simulink model "VTOLAutopilotController"  (R2025a)
settings: configuration reference "VTOLConfiguration" (kept outside this file)
undefined symbols (not defined in the file): Back_Transition_Rate, const, control, controlParams, ControlSampleTime, CriticalTiltAngle, DiscIntNeverNeededParam, dspblkCoreblockFVToolHelper, Fading_time, flightState, FSState, FWControlParams, FWTrimSpeed, gcbh, HoverMission, ReferenceFilterDen, ReferenceFilterNum, tilt_max, tiltIni, TransitioncontrolGains, uavParam, uavParams, VTOLcontrolGains, w_trim, WindDownRate
libraries: simulink x43, slpidlib x35, uavalgslib x7, simulink_extras x1
(part 1 of 8)
settings Model: DataDictionary=VTOLDynamicsData.sldd  PauseTimes=447  Creator=The MathWorks, Inc.  LastModifiedBy=mhcho
settings ConfigSetRef: SourceName=VTOLConfiguration

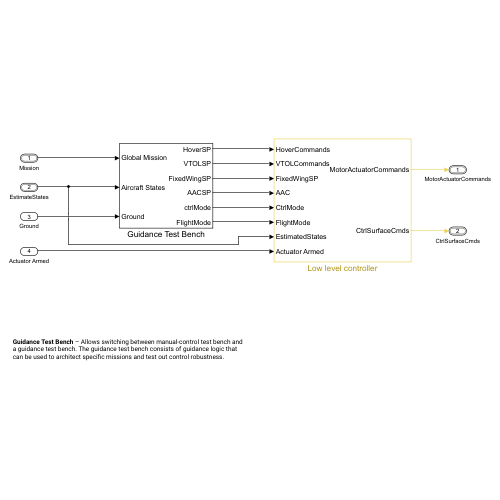
[thumbnail: Simulink's stored preview of the top-level diagram]
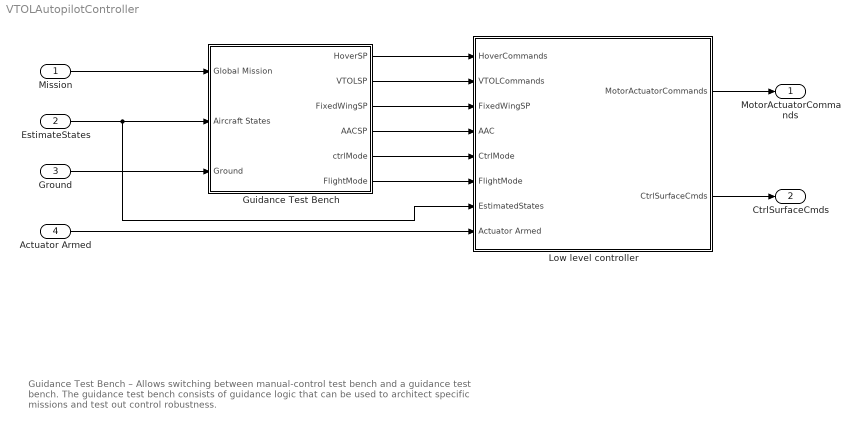
== system VTOLAutopilotController ==
  note: Guidance Test Bench – Allows switching between manual-control test bench and a guidance test bench. The guidance test bench consists of guidance logic that can be used to architect specific missions and test out control robustness.
  Mission : Inport  OutDataTypeStr=Bus: doubleUavPathManager  PortDimensions=length(HoverMission)  SampleTime=0.005  BusOutputAsStruct=on
  EstimateStates : Inport  Port=2  OutDataTypeStr=Bus: stateBus  BusOutputAsStruct=on
  Ground : Inport  Port=3  SampleTime=0.005
  Actuator Armed : Inport  Port=4
  Guidance Test Bench : Subsystem
  Low level controller : Subsystem
  MotorActuatorCommands : Outport  OutDataTypeStr=Bus: RotorCtrlBus  BusOutputAsStruct=on
  CtrlSurfaceCmds : Outport  Port=2  OutDataTypeStr=Bus: FixedWingCtrlBus  BusOutputAsStruct=on
  wires:
  Guidance Test Bench/1(HoverSP) -> Low level controller/1(HoverCommands)
  Guidance Test Bench/4(AACSP) -> Low level controller/4(AAC)
  Guidance Test Bench/6(FlightMode) -> Low level controller/6(FlightMode)
  Guidance Test Bench/5(ctrlMode) -> Low level controller/5(CtrlMode)
  EstimateStates/1 -> Low level controller/7(EstimatedStates), Guidance Test Bench/2(Aircraft States)
  Low level controller/1(MotorActuatorCommands) -> MotorActuatorCommands/1
  Mission/1 -> Guidance Test Bench/1(Global Mission)
  Guidance Test Bench/3(FixedWingSP) -> Low level controller/3(FixedWingSP)
  Low level controller/2(CtrlSurfaceCmds) -> CtrlSurfaceCmds/1
  Ground/1 -> Guidance Test Bench/3(Ground)
  Actuator Armed/1 -> Low level controller/8(Actuator Armed)
  Guidance Test Bench/2(VTOLSP) -> Low level controller/2(VTOLCommands)

== system VTOLAutopilotController/Guidance Test Bench ==
  note: Set control type. In the project shortcut, choose between:
      | 1. Manual control by selecting Manual Mode under Hover and open the subsystem to manually control the UAV in hover mode.
      | 2. Guidance testbench with prebuilt mission by selecting Guidance Mod e in the project shortcut.
  Global Mission : Inport
  Aircraft States : Inport  Port=2
  Ground : Inport  Port=3
  ControlType : Subsystem  Variant=on  VariantControl=Choice
  Variant Subsystem : Subsystem  Variant=on
      settings: PortSchema="{\"entries\":[{\"content\":{\"sides\":[{\"content\":{\"connectorIds\":[\"In1\"]},\"type\":\"ConnectorPlacement.EquallySpacedRectSide\",\"uuid\":\"9fdb7eb7-bc98-4ae8-8dfe-5c3a3cbe5bd4\"},{\"content\":{\"connectorIds\":[\"In2\",\"In3\",\"In4\",\"In5\"],\"side\":\"RIGHT\"},\"type\":\"ConnectorPlacement.EquallySpacedRectSide\",\"uuid\":\"6c20d813-5cc1-435b-898c-bc09e61a7ed0\"},{\"content\":{\"side\":\"TOP\"},\"type\":\"ConnectorPlacement.EquallySpacedRectSide\",\"uuid\":\"a99c14f5-f5c7-4b02-b3e4-43ca7266f03f\"}]},\"type\":\"ConnectorPlacement.EquallySpacedConnector\",\"uuid\":\"e822b786-0a0c-436e-b41c-201e2beca970\"}],\"packageUris\":[\"http://schema.mathworks.com/mf0/Connector/R2020b\"],\"version\":\"1.0\"}"
  HoverSP : Outport
  VTOLSP : Outport  Port=2
  FixedWingSP : Outport  Port=3
  AACSP : Outport  Port=4
  ctrlMode : Outport  Port=5
  FlightMode : Outport  Port=6
  wires:
  ControlType/1(HoverCmds) -> HoverSP/1, Variant Subsystem/2(Position)
  Global Mission/1 -> ControlType/2(Global Mission)
  ControlType/3(FixedWingSP) -> FixedWingSP/1
  ControlType/6(FlightMode) -> Variant Subsystem/5(FlightMode), FlightMode/1
  ControlType/5(CtrlMode) -> Variant Subsystem/4(ControlMode), ctrlMode/1
  ControlType/4(AACSP) -> Variant Subsystem/3(AAC), AACSP/1
  Aircraft States/1 -> Variant Subsystem/1(State), ControlType/1(Aircraft States)
  Ground/1 -> ControlType/3(Ground)
  ControlType/2(VTOLSP) -> VTOLSP/1

== system VTOLAutopilotController/Low level controller ==
  HoverCommands : Inport
  VTOLCommands : Inport  Port=2
  FixedWingSP : Inport  Port=3
  AAC : Inport  Port=4
  CtrlMode : Inport  Port=5
  FlightMode : Inport  Port=6
  EstimatedStates : Inport  Port=7
  Actuator Armed : Inport  Port=8
  Bus Selector : BusSelector  OutputSignals=intransition
  Bus Selector1 : BusSelector  OutputSignals=transitioncondition
  Filter or Estimator : Subsystem
  Fixed Wing Controller : Subsystem  TreatAsAtomicUnit=on  VariantControl=Fixed Wing Controller
  Manual Control : Subsystem
  Multicopter Controller : Subsystem  TreatAsAtomicUnit=on
  Scheduler : Subsystem  SystemSampleTime=0.005
  Tilt Scheduler : Subsystem
  MotorActuatorCommands : Outport
  CtrlSurfaceCmds : Outport  Port=2
  wires:
  EstimatedStates/1 -> Filter or Estimator/1(SensorData)
  [TransitionDone] -> Scheduler/4(TransitionDone)
  Bus Selector1/1 -> [TransitionDone]  "<transitioncondition>"
  Filter or Estimator/1(States) -> Multicopter Controller/3(States), Tilt Scheduler/2(States), Scheduler/5(States), Fixed Wing Controller/1(States)
  Scheduler/1(MotorActuatorCommands) -> MotorActuatorCommands/1
  Scheduler/2(CtrlSurfaceCommands) -> CtrlSurfaceCmds/1
  HoverCommands/1 -> Multicopter Controller/1(HoverCommands)
  Manual Control/1(AERT) -> Fixed Wing Controller/5(AERT)
  Tilt Scheduler/2(FlightState) -> Scheduler/3(FlightState)
  Tilt Scheduler/1(TiltAngle) -> Scheduler/2(TiltSchedule)
  AAC/1 -> Fixed Wing Controller/3(AAC SP)
  CtrlMode/1 -> Bus Selector1/1, Bus Selector/1, Multicopter Controller/4(ControlMode), Fixed Wing Controller/2(Control Mode)
  Actuator Armed/1 -> Scheduler/Enable, Fixed Wing Controller/Enable, Multicopter Controller/Enable
  FixedWingSP/1 -> Fixed Wing Controller/4(FixedWingSP)
  Multicopter Controller/1(MixerCommands) -> Scheduler/1(MotorCommands)
  Fixed Wing Controller/1(Actuator) -> Scheduler/6(FixedWingActuators)
  FlightMode/1 -> [FlightMode]
  [FlightMode] -> Multicopter Controller/5(FlightMode)
  [FlightMode] -> Fixed Wing Controller/6(Flight Mode)
  [FlightMode] -> Tilt Scheduler/1(FlightMode)
  VTOLCommands/1 -> Multicopter Controller/2(VTOLCommands)

== system VTOLAutopilotController/Guidance Test Bench/ControlType ==
  Aircraft States : Inport
  Global Mission : Inport  Port=2
  Ground : Inport  Port=3
  Guidance Testbench : Subsystem  TreatAsAtomicUnit=on  VariantControl=TestMode==1
  Manual Control : Subsystem  TreatAsAtomicUnit=on  VariantControl=TestMode==0
  HoverCmds : Outport
  VTOLSP : Outport  Port=2
  FixedWingSP : Outport  Port=3
  AACSP : Outport  Port=4
  CtrlMode : Outport  Port=5
  FlightMode : Outport  Port=6

== system VTOLAutopilotController/Guidance Test Bench/Variant Subsystem ==
  note: 1) Add Subsystem or Model blocks as valid variant choices.
      | 2) You cannot connect blocks at this level. At simulation, connectivity is automatically
      | determined, based on the active variant and port name matching.
  State : Inport
  Position : Inport  Port=2
  AAC : Inport  Port=3
  ControlMode : Inport  Port=4
  FlightMode : Inport  Port=5
  No-op : Subsystem  VariantControl=Deployment == true
  "Reference Tracking " : Subsystem  VariantControl=Deployment == false

== system VTOLAutopilotController/Low level controller/Filter or Estimator ==
  SensorData : Inport
  States : Outport
  wires:
  SensorData/1 -> States/1

== system VTOLAutopilotController/Low level controller/Fixed Wing Controller ==
  States : Inport
  Control Mode : Inport  Port=2
  AAC SP : Inport  Port=3
  FixedWingSP : Inport  Port=4
  AERT : Inport  Port=5
  Flight Mode : Inport  Port=6
  Enable : EnablePort
  Fixed Wing Controller Module : Subsystem  Variant=on  VariantControl=TuningMode == 0
  Actuator : Outport
  wires:
  States/1 -> Fixed Wing Controller Module/1(States)
  Control Mode/1 -> Fixed Wing Controller Module/2(Control Mode)
  AAC SP/1 -> Fixed Wing Controller Module/3(AAC SP)
  FixedWingSP/1 -> Fixed Wing Controller Module/4(FixedWingSP)
  AERT/1 -> Fixed Wing Controller Module/5(AERT)
  Fixed Wing Controller Module/1(Actuator) -> Actuator/1
  Flight Mode/1 -> Fixed Wing Controller Module/6(Flight Mode)

== system VTOLAutopilotController/Low level controller/Manual Control ==
  Bus Creator : BusCreator  Inputs=4
  Constant{,1..3} (4 alike) : Constant  Value=0  SampleTime=-1
  AERT : Outport
  wires:
  Constant/1 -> Bus Creator/1  "aileron"
  Constant1/1 -> Bus Creator/2  "throttle"
  Constant2/1 -> Bus Creator/3  "elevator"
  Constant3/1 -> Bus Creator/4  "rudder"
  Bus Creator/1 -> AERT/1

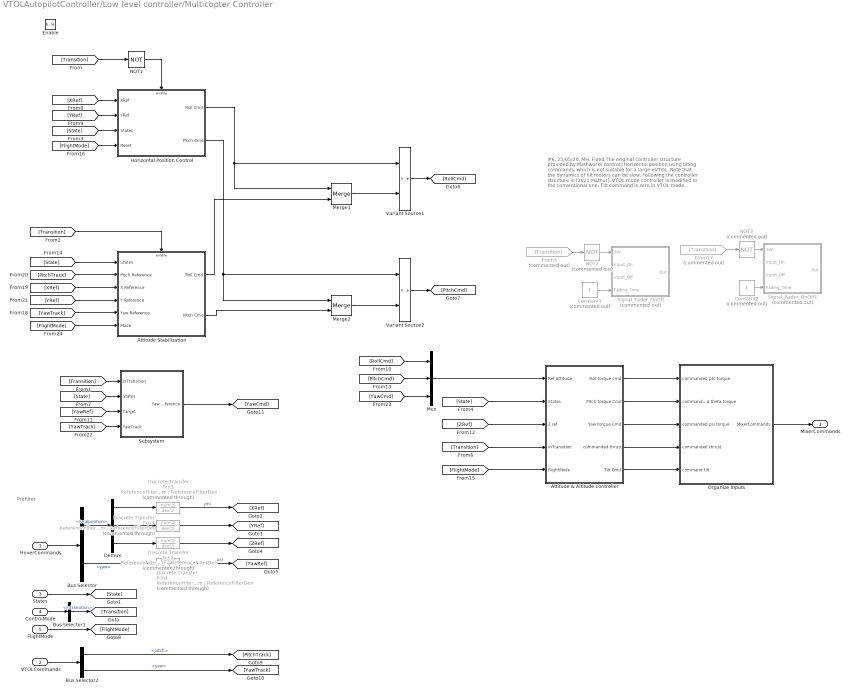
== system VTOLAutopilotController/Low level controller/Multicopter Controller ==
  note: Prefilter
  note: #6, 25/05/20, MH, Fixed
      | The original controller structure provided by
      | Mathworks controls horizontal position using
      | tilting commands, which is not suitable for
      | a large eVTOL. Note that the dynamics of tilt
      | motors can be slow. Following the controller
      | structure in [2021 Mathur], VTOL mode controller
      | is modified to the conventional one.
      | Tilt command is zero in VTOL mode.
  HoverCommands : Inport
  VTOLCommands : Inport  Port=2
  States : Inport  Port=3
  ControlMode : Inport  Port=4
  FlightMode : Inport  Port=5
  Enable : EnablePort
  Attitude & Altitude controller : Subsystem
  Attitude Stabilization : Subsystem  TreatAsAtomicUnit=on
  Bus Selector : BusSelector  OutputSignals=localposition,yaw
  Bus Selector1 : BusSelector  OutputSignals=intransition
  Bus Selector2 : BusSelector  OutputSignals=pitch,yaw
  Constant1 : Constant  Commented=on
  Constant2 : Constant  Commented=on
  Demux : Demux  Outputs=3
  Discrete Transfer Fcn1 : DiscreteTransferFcn  Commented=through  LoadFcn=dspblkCoreblockFVToolHelper(gcbh,'load');  Numerator=ReferenceFilterNum  Denominator=ReferenceFilterDen
      settings: CopyFcn=dspblkCoreblockFVToolHelper(gcbh,'copy');  DeleteFcn=dspblkCoreblockFVToolHelper(gcbh,'close');  ModelCloseFcn=dspblkCoreblockFVToolHelper(gcbh,'close');  PreSaveFcn=dspblkCoreblockFVToolHelper(gcbh,'presave');  PostSaveFcn=dspblkCoreblockFVToolHelper(gcbh,'postsave');  CloseFcn=dspblkCoreblockFVToolHelper(gcbh,'close');
  Discrete Transfer Fcn2 : DiscreteTransferFcn  Commented=through  Numerator=ReferenceFilterNum  Denominator=ReferenceFilterDen
  Discrete Transfer Fcn3 : DiscreteTransferFcn  Commented=through  LoadFcn=dspblkCoreblockFVToolHelper(gcbh,'load');  Numerator=ReferenceFilterNum  Denominator=ReferenceFilterDen
      settings: CopyFcn=dspblkCoreblockFVToolHelper(gcbh,'copy');  DeleteFcn=dspblkCoreblockFVToolHelper(gcbh,'close');  ModelCloseFcn=dspblkCoreblockFVToolHelper(gcbh,'close');  PreSaveFcn=dspblkCoreblockFVToolHelper(gcbh,'presave');  PostSaveFcn=dspblkCoreblockFVToolHelper(gcbh,'postsave');  CloseFcn=dspblkCoreblockFVToolHelper(gcbh,'close');
  Discrete Transfer Fcn4 : DiscreteTransferFcn  Commented=through  Numerator=ReferenceFilterNum  Denominator=ReferenceFilterDen
  From17 : From  Commented=on  GotoTag=Transition
  From5 : From  Commented=on  GotoTag=Transition
  Horizontal Position Control : Subsystem  TreatAsAtomicUnit=on
  Merge1 : Merge
  Merge2 : Merge
  Mux : Mux  Inputs=3
  NOT1 : Logic  Operator=NOT  IconShape=distinctive  AllPortsSameDT=off  OutDataTypeStr=boolean
  NOT2 : Logic  Commented=on  Operator=NOT  IconShape=distinctive  AllPortsSameDT=off  OutDataTypeStr=boolean
  NOT3 : Logic  Commented=on  Operator=NOT  IconShape=distinctive  AllPortsSameDT=off  OutDataTypeStr=boolean
  Organize Inputs : Subsystem
  Signal_Fader_OnOff : Subsystem  Commented=on
  Signal_Fader_OnOff1 : Subsystem  Commented=on
  Subsystem : Subsystem
  Variant Source1 : VariantSource  VariantControls={TuningMode~=0, TuningMode==0}
  Variant Source2 : VariantSource  VariantControls={TuningMode~=0, TuningMode==0}
  MixerCommands : Outport
  wires:
  Organize Inputs/1(MixerCommands) -> MixerCommands/1
  [State] -> Subsystem/2(States)
  Discrete Transfer Fcn4/1 -> [YRef]
  [State] -> Horizontal Position Control/3(States)
  [YawRef] -> Subsystem/3(Target)
  [Transition] -> Subsystem/1(inTransition)
  Horizontal Position Control/1(Roll Cmd) -> Merge1/1, Variant Source1/1
  [Transition] -> Attitude Stabilization/Enable
  NOT1/1 -> Horizontal Position Control/Enable
  Discrete Transfer Fcn2/1 -> [ZRef]
  [XRef] -> Horizontal Position Control/1(XRef)
  [YRef] -> Horizontal Position Control/2(YRef)
  States/1 -> [State]
  HoverCommands/1 -> Bus Selector/1
  Mux/1 -> Attitude & Altitude controller/1(Ref Attitude)
  [State] -> Attitude & Altitude controller/2(States)
  [ZRef] -> Attitude & Altitude controller/3(Z ref)
  [Transition] -> Attitude & Altitude controller/4(InTransition)
  Attitude & Altitude controller/1(Roll torque cmd) -> Organize Inputs/1(commanded phi torque)
  Attitude & Altitude controller/2(Pitch torque Cmd) -> Organize Inputs/2(commanded theta torque)
  Attitude & Altitude controller/4(commanded thrust) -> Organize Inputs/4(commanded thrust)
  Discrete Transfer Fcn3/1 -> [XRef]  "phi"
  Attitude & Altitude controller/3(Yaw torque Cmd) -> Organize Inputs/3(commanded psi torque)
  [Transition] -> NOT1/1
  Horizontal Position Control/2(Pitch Cmd) -> Merge2/1, Variant Source2/1
  Variant Source1/1 -> [RollCmd]
  Variant Source2/1 -> [PitchCmd]
  [RollCmd] -> Mux/1
  [PitchCmd] -> Mux/2
  [State] -> Attitude Stabilization/1(States)
  From5/1 -> NOT2/1
  NOT2/1 -> Signal_Fader_OnOff/1(SW)
  Constant1/1 -> Signal_Fader_OnOff/4(Fading_Time)
  FlightMode/1 -> [FlightMode]
  [FlightMode] -> Attitude & Altitude controller/5(FlightMode)
  NOT3/1 -> Signal_Fader_OnOff1/1(SW)
  From17/1 -> NOT3/1
  Constant2/1 -> Signal_Fader_OnOff1/4(Fading_Time)
  [FlightMode] -> Horizontal Position Control/4(Reset)
  Attitude & Altitude controller/5(Tilt Cmd) -> Organize Inputs/5(command tilt)
  Demux/1 -> Discrete Transfer Fcn3/1
  Demux/2 -> Discrete Transfer Fcn4/1
  Demux/3 -> Discrete Transfer Fcn2/1
  Bus Selector/2 -> Discrete Transfer Fcn1/1  "<yaw>"
  Bus Selector/1 -> Demux/1  "<localposition>"
  Attitude Stabilization/1(Roll Cmd) -> Merge1/2
  Merge1/1 -> Variant Source1/2
  Attitude Stabilization/2(Pitch Cmd) -> Merge2/2
  Merge2/1 -> Variant Source2/2
  ControlMode/1 -> Bus Selector1/1
  Bus Selector1/1 -> [Transition]  "<intransition>"
  VTOLCommands/1 -> Bus Selector2/1
  Bus Selector2/1 -> [PitchTrack]  "<pitch>"
  [PitchTrack] -> Attitude Stabilization/2(Pitch Reference)
  Bus Selector2/2 -> [YawTrack]  "<yaw>"
  Discrete Transfer Fcn1/1 -> [YawRef]  "psi"
  [YawTrack] -> Attitude Stabilization/5(Yaw Reference)
  [XRef] -> Attitude Stabilization/3(X Reference)
  [YRef] -> Attitude Stabilization/4(Y Reference)
  [YawTrack] -> Subsystem/4(YawTrack)
  Subsystem/1(Yaw Reference) -> [YawCmd]
  [YawCmd] -> Mux/3
  [FlightMode] -> Attitude Stabilization/6(Mode)

== system VTOLAutopilotController/Low level controller/Scheduler ==
  MotorCommands : Inport
  TiltSchedule : Inport  Port=2
  FlightState : Inport  Port=3  OutDataTypeStr=Enum: flightState
  TransitionDone : Inport  Port=4
  States : Inport  Port=5
  FixedWingActuators : Inport  Port=6
  Enable : EnablePort
  FixedWingScheduler : Subsystem
  Subsystem : Subsystem
  To Workspace1 : ToWorkspace  VariableName=Flight_Mode  SaveFormat=Timeseries  SampleTime=-1
  MotorActuatorCommands : Outport  OutputWhenDisabled=reset  InitialOutput=0
  CtrlSurfaceCommands : Outport  Port=2  OutDataTypeStr=Bus: FixedWingCtrlBus  OutputWhenDisabled=reset  InitialOutput=0  VectorParamsAs1DForOutWhenUnconnected=off
  wires:
  FixedWingScheduler/1(ActuatorControls) -> Subsystem/2(FixedWingActuators), CtrlSurfaceCommands/1
  FlightState/1 -> FixedWingScheduler/1(FlightState), [FlightState], To Workspace1/1
  TiltSchedule/1 -> Subsystem/4(TiltSchedule)
  Subsystem/1(ActuatorControls) -> MotorActuatorCommands/1
  MotorCommands/1 -> Subsystem/3(MotorCommands)
  FixedWingActuators/1 -> FixedWingScheduler/2(FixedWingActuators)
  TransitionDone/1 -> FixedWingScheduler/3(TransitionDone), [TransitionDone]
  States/1 -> FixedWingScheduler/4(States), Subsystem/6(States)
  [FlightState] -> Subsystem/1(FlightState)
  [TransitionDone] -> Subsystem/5(TransitionDone)

== system VTOLAutopilotController/Low level controller/Tilt Scheduler ==
  note: Forward Transition Tilt Mode Manager
  note: Back Transition Tilt Mode Manager
  FlightMode : Inport
  States : Inport  Port=2
  Back Transition Scheduler : Subsystem
  Forward Transition Scheduler : Subsystem
  TiltAngle : Outport
  FlightState : Outport  Port=2
  wires:
  States/1 -> Back Transition Scheduler/3(States)
  Back Transition Scheduler/1(TiltAngle) -> TiltAngle/1
  FlightMode/1 -> Back Transition Scheduler/2(FlightMode), Forward Transition Scheduler/1(FlightMode)
  Forward Transition Scheduler/1(FlightState) -> FlightState/1
  Forward Transition Scheduler/2(Tilt Schedule) -> Back Transition Scheduler/1(Tilt Schedule)

== system VTOLAutopilotController/Guidance Test Bench/ControlType/Guidance Testbench ==
  Global Mission : Inport
  Aircraft States : Inport  Port=2
  Ground : Inport  Port=3
  Control Rate Transition : Subsystem
  Guidance Logic : Subsystem  VariantControl=guidanceType==1
  HoverCmds : Outport
  VTOLSP : Outport  Port=2
  FixedWingSP : Outport  Port=3
  AACSP : Outport  Port=4
  CtrlMode : Outport  Port=5
  FlightMode : Outport  Port=6
  wires:
  Aircraft States/1 -> Guidance Logic/1(UAVState)
  Global Mission/1 -> Guidance Logic/2(GCSCommands)
  Guidance Logic/1(HoverSP) -> Control Rate Transition/1("HoverSP ")
  Control Rate Transition/1(hoverSP) -> HoverCmds/1
  Ground/1 -> Guidance Logic/3(Ground)
  Guidance Logic/2(VTOLSP) -> Control Rate Transition/2(VTOLSP)
  Guidance Logic/3(FixedWingSP) -> Control Rate Transition/3(FixedWingSP)
  Guidance Logic/4(AACSP) -> Control Rate Transition/4(AACSP)
  Guidance Logic/5(CtrlMode) -> Control Rate Transition/5(CtrlMode)
  Guidance Logic/6(FlightMode) -> Control Rate Transition/6(FlightMode)
  Control Rate Transition/2(vtolSP) -> VTOLSP/1
  Control Rate Transition/3(fixedwingSP) -> FixedWingSP/1
  Control Rate Transition/4(aacSP) -> AACSP/1
  Control Rate Transition/5(ctrlMode) -> CtrlMode/1
  Control Rate Transition/6(flightMode) -> FlightMode/1

== system VTOLAutopilotController/Guidance Test Bench/ControlType/Manual Control ==
  Global Mission : Inport
  Aircraft States : Inport  Port=2
  Command Interface : Subsystem
  HoverCmds : Outport
  FixedWingSP : Outport  Port=2
  AACSP : Outport  Port=3
  CtrlMode : Outport  Port=4
  FlightMode : Outport  Port=5
  wires:
  Global Mission/1 -> Command Interface/1(Global Mission)
  Aircraft States/1 -> Command Interface/2(Aircraft States)
  Command Interface/1(ctrlMode) -> CtrlMode/1
  Command Interface/2(FixedWingSP) -> FixedWingSP/1
  Command Interface/3(AACSP) -> AACSP/1
  Command Interface/4(PositionCmds) -> HoverCmds/1
  Command Interface/5(FlightMode) -> FlightMode/1

== system VTOLAutopilotController/Guidance Test Bench/Variant Subsystem/No-op ==
  State : Inport
  Terminator : Terminator
  wires:
  State/1 -> Terminator/1

== system VTOLAutopilotController/Guidance Test Bench/Variant Subsystem/Reference Tracking  ==
  State : Inport
  Position : Inport  Port=2
  AAC : Inport  Port=3
  ControlMode : Inport  Port=4
  FlightMode : Inport  Port=5
  Bus Creator : BusCreator  Inputs=8
  Bus Selector : BusSelector  OutputSignals=lateralguidance,airspeedaltitude,attitude,manual,armed,intransition,transitioncondition
  Data Type Conversion : DataTypeConversion  OutDataTypeStr=uint8  SaturateOnIntegerOverflow=off  RndMeth=Floor
  Fixed Wing Reference : Subsystem
  Hover Reference : Subsystem
  To Workspace1 : ToWorkspace  VariableName=GuidanceFeedback  SaveFormat=Structure With Time  SampleTime=-1
  Transition Reference : Subsystem
  wires:
  State/1 -> Transition Reference/1(States), Fixed Wing Reference/2(States), Hover Reference/2(Position Reference)
  AAC/1 -> Fixed Wing Reference/1(AAC Commands)
  Position/1 -> Hover Reference/1(Position Command)
  ControlMode/1 -> Bus Selector/1
  Bus Selector/7 -> Bus Creator/7  "<transitioncondition>"
  Bus Selector/6 -> Bus Creator/6  "<intransition>"
  Bus Selector/5 -> Bus Creator/5  "<armed>"
  Bus Selector/4 -> Bus Creator/4  "<manual>"
  Bus Selector/1 -> Bus Creator/1  "<lateralguidance>"
  Bus Creator/1 -> To Workspace1/1
  FlightMode/1 -> Data Type Conversion/1
  Data Type Conversion/1 -> Bus Creator/8  "FlightMode"
  Bus Selector/2 -> Bus Creator/2  "<airspeedaltitude>"
  Bus Selector/3 -> Bus Creator/3  "<attitude>"

== system VTOLAutopilotController/Low level controller/Fixed Wing Controller/Fixed Wing Controller Module ==
  States : Inport
  Control Mode : Inport  Port=2
  AAC SP : Inport  Port=3
  FixedWingSP : Inport  Port=4
  AERT : Inport  Port=5
  Flight Mode : Inport  Port=6
  Fixed Wing Controller Simulation : Subsystem  VariantControl=TuningMode == 0
  Fixed Wing Controller Tuning : Subsystem  VariantControl=TuningMode==1
  Actuator : Outport

== system VTOLAutopilotController/Low level controller/Multicopter Controller/Attitude & Altitude controller ==
  Ref Attitude : Inport
  States : Inport  Port=2
  Z ref : Inport  Port=3
  InTransition : Inport  Port=4
  FlightMode : Inport  Port=5
  Altitude Control : Subsystem
  Derivative Gain : Subsystem  VariantControl=AttitudeControl==1
  Roll torque cmd : Outport
  Pitch torque Cmd : Outport  Port=2
  Yaw torque Cmd : Outport  Port=3
  commanded thrust : Outport  Port=4
  Tilt Cmd : Outport  Port=5
  wires:
  Altitude Control/1(commanded thrust) -> commanded thrust/1
  Derivative Gain/1(Roll torque cmd) -> Roll torque cmd/1
  InTransition/1 -> Derivative Gain/3(InTransition), Altitude Control/3(InTransition)
  Derivative Gain/2(Pitch torque Cmd) -> Pitch torque Cmd/1
  States/1 -> Altitude Control/1(States), Derivative Gain/2(States)
  Derivative Gain/3(Yaw torque Cmd) -> Yaw torque Cmd/1
  Z ref/1 -> Altitude Control/2(Z ref)
  FlightMode/1 -> Derivative Gain/4(Reset), Altitude Control/4(FlightMode)
  Ref Attitude/1 -> Derivative Gain/1(Ref Attitude)
  Derivative Gain/4(Tilt Cmd) -> Tilt Cmd/1

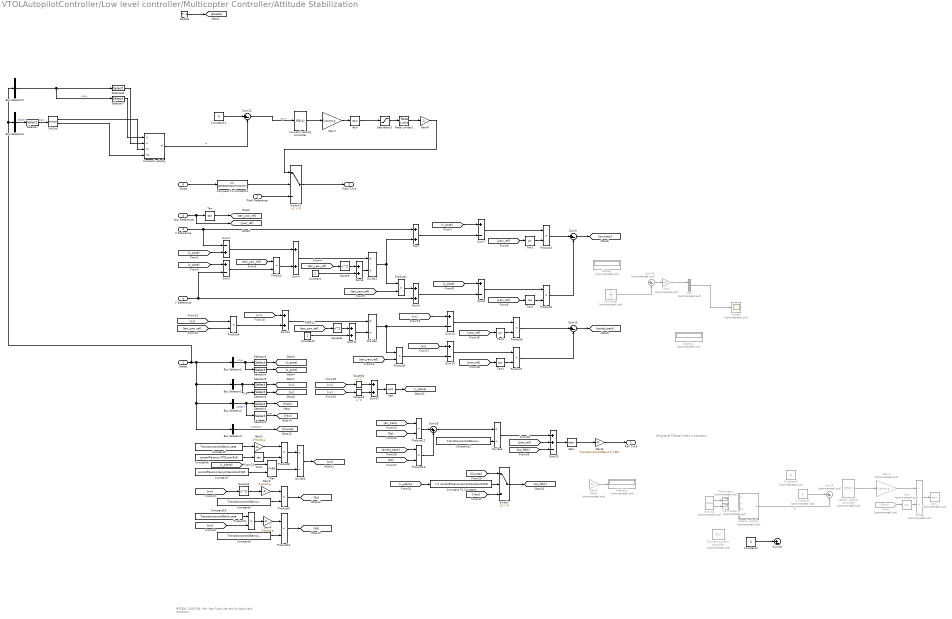
== system VTOLAutopilotController/Low level controller/Multicopter Controller/Attitude Stabilization ==
  note: Wing-level Tiltrotor when in transition.
  note: #TODO, 25/07/05, MH, Not Fixed
      | Use this for backward transition.
  States : Inport
  Pitch Reference : Inport  Port=2
  X Reference : Inport  Port=3
  Y Reference : Inport  Port=4
  Yaw Reference : Inport  Port=5
  Mode : Inport  Port=6
  Enable : EnablePort  ShowOutputPort=on
  Asin : Trigonometry  Operator=asin
  Asin1 : Trigonometry  Commented=on  Operator=asin
  Atan : Trigonometry  Operator=atan
  Bus Selector1 : BusSelector  OutputSignals=Ve
  Bus Selector2 : BusSelector  OutputSignals=Euler
  Bus Selector3 : BusSelector  OutputSignals=Xe
  Bus Selector4 : BusSelector  OutputSignals=course
  Bus Selector5 : BusSelector  OutputSignals=Ve
  Bus Selector6 : BusSelector  OutputSignals=Euler
  Compare To Constant : simulink/Logic and Bit Operations/Compare To Constant  relop=>=  const=controlParams.tempVtransitionFWD  OutDataTypeStr=boolean
  Compare To Constant1 : simulink/Logic and Bit Operations/Compare To Constant  relop===  const=flightState.BackTransition  OutDataTypeStr=boolean
  Constant : Constant
  Constant1 : Constant  Commented=on  Value=0
  Constant10 : Constant  Value=TransitioncontrolGains.zeta
  Constant11 : Constant  Value=0
  Constant12 : Constant  Value=TransitioncontrolGains.L
  Constant2 : Constant  Value=0
  Constant3 : Constant
  Constant4 : Constant  Commented=on  Value=0
  Constant5 : Constant  Value=TransitioncontrolGains.zeta
  Constant6 : Constant  Value=controlParams.VTOLmaxRoll
  Constant7 : Constant  Value=controlParams.tempVtransitionFWD
  Constant8 : Constant  Value=TransitioncontrolGains.L
  Constant9 : Constant  Value=TransitioncontrolGains.L
  Cos : Trigonometry  Commented=on  Operator=cos
  Display : Display  Commented=on
  Display1 : Display  Commented=on
  Display2 : Display  Commented=on
  Divide : Product  Commented=on  Inputs=*/
  Divide{1..4} (4 alike) : Product  Inputs=*/
  Forward position controller : slpidlib/PID Controller  Commented=on  Controller=P  Form=Parallel  TimeDomain=Discrete-time  UseExternalTs=off  SampleTime=-1  IntegratorMethod=Forward Euler  FilterMethod=Forward Euler  ControllerParametersSource=internal  P=VTOLcontrolGains.P_X  I=controlParams.I_X  UseKiTs=off  D=0.741088334151374  UseExternalDerivativeSource=off  N=1.14081860742283  UseFilter=on  TunerSelectOption=Transfer Function Based (PID Tuner App)  InitialConditionSource=internal  InitialConditionForIntegrator=0  InitialConditionForFilter=0  DifferentiatorICPrevScaledInput=0  ExternalReset=none  TrackingMode=off  Kt=1  LimitOutput=off  SatLimitsSource=internal  UpperSaturationLimit=inf  LowerSaturationLimit=-inf  LinearizeAsGain=on  AntiWindupMode=none  Kb=1  LimitIntegrator=off  UpperIntegratorSaturationLimit=inf  LowerIntegratorSaturationLimit=-inf  POutMin=[]  POutMax=[]  IOutMin=[]  IOutMax=[]  DOutMin=[]  DOutMax=[]  NOutMin=[]  NOutMax=[]  SumOutMin=[]  SumOutMax=[]  SaturationOutMin=[]  SaturationOutMax=[]  PParamMin=[]  PParamMax=[]  IParamMin=[]  IParamMax=[]  DParamMin=[]  DParamMax=[]  NParamMin=[]  NParamMax=[]  KbParamMin=[]  KbParamMax=[]  KtParamMin=[]  KtParamMax=[]  KbOutMin=[]  KbOutMax=[]  KtOutMin=[]  KtOutMax=[]  IntegratorOutMin=[]  IntegratorOutMax=[]  FilterOutMin=[]  FilterOutMax=[]  SumI1OutMin=[]  SumI1OutMax=[]  SumI2OutMin=[]  SumI2OutMax=[]  SumI3OutMin=[]  SumI3OutMax=[]  SumI4OutMin=[]  SumI4OutMax=[]  SumDOutMin=[]  SumDOutMax=[]  DifferentiatorOutMin=[]  DifferentiatorOutMax=[]  FilterDiffOutCoefMin=[]  FilterDiffOutCoefMax=[]  ReciprocalOutMin=[]  ReciprocalOutMax=[]  SumDenOutMin=[]  SumDenOutMax=[]  SumNumOutMin=[]  SumNumOutMax=[]  DivideOutMin=[]  DivideOutMax=[]  UdiffTsProdOutMin=[]  UdiffTsProdOutMax=[]  NTsProdOutMin=[]  NTsProdOutMax=[]  UintegralTsProdOutMin=[]  UintegralTsProdOutMax=[]  UngainTsProdOutMin=[]  UngainTsProdOutMax=[]  ClampingZeroOutDataTypeStr=Inherit: Inherit via back propagation  ClampingZeroOutMin=[]  ClampingZeroOutMax=[]  FilterDenConstantOutDataTypeStr=Inherit: Inherit via back propagation  FilterDenConstantOutMin=[]  FilterDenConstantOutMax=[]  PCopyOutDataTypeStr=Inherit: Inherit via back propagation  PCopyOutMin=[]  PCopyOutMax=[]  NCopyOutDataTypeStr=Inherit: Inherit via back propagation  NCopyOutMin=[]  NCopyOutMax=[]  IntegratorContinuousStateAttributes=''  IntegratorStateMustResolveToSignalObject=off  IntegratorRTWStateStorageClass=Auto  FilterContinuousStateAttributes=''  FilterStateMustResolveToSignalObject=off  FilterRTWStateStorageClass=Auto  ParallelPVariant=InternalParameters  IdealPVariant=Disabled  IVariant=Disabled  DVariant=Disabled  IntegratorVariant=Disabled  SatVariant=Disabled  AWVariant=Disabled  PCopyVariant=Disabled  TRVariant=Disabled  FdbkBlocksVariant=Forward  IdealPFdbkVariant=Disabled  SatFdbkVariant=Disabled  DerivativeFilterVariant=Disabled  NVariant=Disabled  NCopyVariant=Disabled_SignalSpec  FilterICVariant=Disabled  IntegratorICVariant=Disabled  ExternalResetVariant=Disabled  TRSumVariant=Passthrough  SumFdbkVariant=Disabled  SumVariant=Passthrough_P  TsampFilterVariant=InternalTs  TsampNgainVariant=Passthrough  TsampIntegralVariant=Disabled_SignalSpec  ExternalSaturationOutDataTypeStr=Inherit: Same as second input  DerivativeSourceVariant=Disabled  PreIntVariant=InternalPreInt
  Forward velocity : Subsystem
  Forward velocity controller : slpidlib/PID Controller  Controller=PD  Form=Parallel  TimeDomain=Discrete-time  UseExternalTs=off  SampleTime=-1  IntegratorMethod=Forward Euler  FilterMethod=Forward Euler  ControllerParametersSource=internal  P=VTOLcontrolGains.P_VX*0.2  I=VTOLcontrolGains.I_VX  UseKiTs=off  D=VTOLcontrolGains.D_VX*0.2  UseExternalDerivativeSource=off  N=VTOLcontrolGains.N_VX  UseFilter=on  TunerSelectOption=Transfer Function Based (PID Tuner App)  InitialConditionSource=internal  InitialConditionForIntegrator=0  InitialConditionForFilter=0  DifferentiatorICPrevScaledInput=0  ExternalReset=none  TrackingMode=off  Kt=1  LimitOutput=off  SatLimitsSource=internal  UpperSaturationLimit=inf  LowerSaturationLimit=-inf  LinearizeAsGain=on  AntiWindupMode=none  Kb=1  LimitIntegrator=off  UpperIntegratorSaturationLimit=inf  LowerIntegratorSaturationLimit=-inf  POutMin=[]  POutMax=[]  IOutMin=[]  IOutMax=[]  DOutMin=[]  DOutMax=[]  NOutMin=[]  NOutMax=[]  SumOutMin=[]  SumOutMax=[]  SaturationOutMin=[]  SaturationOutMax=[]  PParamMin=[]  PParamMax=[]  IParamMin=[]  IParamMax=[]  DParamMin=[]  DParamMax=[]  NParamMin=[]  NParamMax=[]  KbParamMin=[]  KbParamMax=[]  KtParamMin=[]  KtParamMax=[]  KbOutMin=[]  KbOutMax=[]  KtOutMin=[]  KtOutMax=[]  IntegratorOutMin=[]  IntegratorOutMax=[]  FilterOutMin=[]  FilterOutMax=[]  SumI1OutMin=[]  SumI1OutMax=[]  SumI2OutMin=[]  SumI2OutMax=[]  SumI3OutMin=[]  SumI3OutMax=[]  SumI4OutMin=[]  SumI4OutMax=[]  SumDOutMin=[]  SumDOutMax=[]  DifferentiatorOutMin=[]  DifferentiatorOutMax=[]  FilterDiffOutCoefMin=[]  FilterDiffOutCoefMax=[]  ReciprocalOutMin=[]  ReciprocalOutMax=[]  SumDenOutMin=[]  SumDenOutMax=[]  SumNumOutMin=[]  SumNumOutMax=[]  DivideOutMin=[]  DivideOutMax=[]  UdiffTsProdOutMin=[]  UdiffTsProdOutMax=[]  NTsProdOutMin=[]  NTsProdOutMax=[]  UintegralTsProdOutMin=[]  UintegralTsProdOutMax=[]  UngainTsProdOutMin=[]  UngainTsProdOutMax=[]  ClampingZeroOutDataTypeStr=Inherit: Inherit via back propagation  ClampingZeroOutMin=[]  ClampingZeroOutMax=[]  FilterDenConstantOutDataTypeStr=Inherit: Inherit via back propagation  FilterDenConstantOutMin=[]  FilterDenConstantOutMax=[]  PCopyOutDataTypeStr=Inherit: Inherit via back propagation  PCopyOutMin=[]  PCopyOutMax=[]  NCopyOutDataTypeStr=Inherit: Inherit via back propagation  NCopyOutMin=[]  NCopyOutMax=[]  IntegratorContinuousStateAttributes=''  IntegratorStateMustResolveToSignalObject=off  IntegratorRTWStateStorageClass=Auto  FilterContinuousStateAttributes=''  FilterStateMustResolveToSignalObject=off  FilterRTWStateStorageClass=Auto  ParallelPVariant=InternalParameters  IdealPVariant=Disabled  IVariant=Disabled  DVariant=InternalParameters  IntegratorVariant=Disabled  SatVariant=Disabled  AWVariant=Disabled  PCopyVariant=Disabled  TRVariant=Disabled  FdbkBlocksVariant=Forward  IdealPFdbkVariant=Disabled  SatFdbkVariant=Disabled  DerivativeFilterVariant=ForwardEulerFilter  NVariant=InternalParameters  NCopyVariant=Disabled  FilterICVariant=InternalICsFilter  IntegratorICVariant=Disabled  ExternalResetVariant=Disabled  TRSumVariant=Passthrough  SumFdbkVariant=Disabled  SumVariant=Sum_PD  TsampFilterVariant=InternalTs  TsampNgainVariant=Passthrough  TsampIntegralVariant=Disabled_SignalSpec  ExternalSaturationOutDataTypeStr=Inherit: Same as second input  DerivativeSourceVariant=ErrorSignal  PreIntVariant=InternalPreInt
  From : From  Commented=on  GotoTag=Pitch
  Gain : Gain  Commented=on  Gain=200
  Gain1 : Gain  Commented=on  Gain=1/const.g
  Gain2 : Gain  Gain=2*const.g
  Gain3 : Gain  Gain=1/const.g
  Gain4 : Gain  Gain=2/const.g
  Gain5 : Gain  Commented=on  Gain=180/pi
  Gain6 : Gain  Gain=TransitioncontrolGains.P_YAW
  Gain7 : Gain  Gain=1/const.g
  Gain8 : Gain  Gain=-1
  Lateral velocity : Subsystem  Commented=on
  "Lateral velocity controller " : slpidlib/PID Controller  Commented=on  Controller=PD  Form=Parallel  TimeDomain=Discrete-time  UseExternalTs=off  SampleTime=-1  IntegratorMethod=Forward Euler  FilterMethod=Forward Euler  ControllerParametersSource=internal  P=VTOLcontrolGains.P_VY  I=VTOLcontrolGains.I_VY  UseKiTs=off  D=VTOLcontrolGains.D_VY  UseExternalDerivativeSource=off  N=VTOLcontrolGains.N_VY  UseFilter=on  TunerSelectOption=Transfer Function Based (PID Tuner App)  InitialConditionSource=internal  InitialConditionForIntegrator=0  InitialConditionForFilter=0  DifferentiatorICPrevScaledInput=0  ExternalReset=none  TrackingMode=off  Kt=1  LimitOutput=off  SatLimitsSource=internal  UpperSaturationLimit=inf  LowerSaturationLimit=-inf  LinearizeAsGain=on  AntiWindupMode=none  Kb=1  LimitIntegrator=off  UpperIntegratorSaturationLimit=inf  LowerIntegratorSaturationLimit=-inf  POutMin=[]  POutMax=[]  IOutMin=[]  IOutMax=[]  DOutMin=[]  DOutMax=[]  NOutMin=[]  NOutMax=[]  SumOutMin=[]  SumOutMax=[]  SaturationOutMin=[]  SaturationOutMax=[]  PParamMin=[]  PParamMax=[]  IParamMin=[]  IParamMax=[]  DParamMin=[]  DParamMax=[]  NParamMin=[]  NParamMax=[]  KbParamMin=[]  KbParamMax=[]  KtParamMin=[]  KtParamMax=[]  KbOutMin=[]  KbOutMax=[]  KtOutMin=[]  KtOutMax=[]  IntegratorOutMin=[]  IntegratorOutMax=[]  FilterOutMin=[]  FilterOutMax=[]  SumI1OutMin=[]  SumI1OutMax=[]  SumI2OutMin=[]  SumI2OutMax=[]  SumI3OutMin=[]  SumI3OutMax=[]  SumI4OutMin=[]  SumI4OutMax=[]  SumDOutMin=[]  SumDOutMax=[]  DifferentiatorOutMin=[]  DifferentiatorOutMax=[]  FilterDiffOutCoefMin=[]  FilterDiffOutCoefMax=[]  ReciprocalOutMin=[]  ReciprocalOutMax=[]  SumDenOutMin=[]  SumDenOutMax=[]  SumNumOutMin=[]  SumNumOutMax=[]  DivideOutMin=[]  DivideOutMax=[]  UdiffTsProdOutMin=[]  UdiffTsProdOutMax=[]  NTsProdOutMin=[]  NTsProdOutMax=[]  UintegralTsProdOutMin=[]  UintegralTsProdOutMax=[]  UngainTsProdOutMin=[]  UngainTsProdOutMax=[]  ClampingZeroOutDataTypeStr=Inherit: Inherit via back propagation  ClampingZeroOutMin=[]  ClampingZeroOutMax=[]  FilterDenConstantOutDataTypeStr=Inherit: Inherit via back propagation  FilterDenConstantOutMin=[]  FilterDenConstantOutMax=[]  PCopyOutDataTypeStr=Inherit: Inherit via back propagation  PCopyOutMin=[]  PCopyOutMax=[]  NCopyOutDataTypeStr=Inherit: Inherit via back propagation  NCopyOutMin=[]  NCopyOutMax=[]  IntegratorContinuousStateAttributes=''  IntegratorStateMustResolveToSignalObject=off  IntegratorRTWStateStorageClass=Auto  FilterContinuousStateAttributes=''  FilterStateMustResolveToSignalObject=off  FilterRTWStateStorageClass=Auto  ParallelPVariant=InternalParameters  IdealPVariant=Disabled  IVariant=Disabled  DVariant=InternalParameters  IntegratorVariant=Disabled  SatVariant=Disabled  AWVariant=Disabled  PCopyVariant=Disabled  TRVariant=Disabled  FdbkBlocksVariant=Forward  IdealPFdbkVariant=Disabled  SatFdbkVariant=Disabled  DerivativeFilterVariant=ForwardEulerFilter  NVariant=InternalParameters  NCopyVariant=Disabled  FilterICVariant=InternalICsFilter  IntegratorICVariant=Disabled  ExternalResetVariant=Disabled  TRSumVariant=Passthrough  SumFdbkVariant=Disabled  SumVariant=Sum_PD  TsampFilterVariant=InternalTs  TsampNgainVariant=Passthrough  TsampIntegralVariant=Disabled_SignalSpec  ExternalSaturationOutDataTypeStr=Inherit: Same as second input  DerivativeSourceVariant=ErrorSignal  PreIntVariant=InternalPreInt
  Max : MinMax  Function=max  Inputs=2
  Mux : Mux  Commented=on  Inputs=2
  Product{,1..13} (14 alike) : Product
  Rate Limiter1 : RateLimiter  RisingSlewLimit=controlParams.VTOLmaxPitchSlewrate  FallingSlewLimit=controlParams.VTOLminPitchSlewrate  SampleTimeMode=inherited
  Saturation1 : Saturate  UpperLimit=controlParams.VTOLmaxPitch  LowerLimit=controlParams.VTOLminPitch
  Scope : Scope  Commented=on
      settings: ActiveDisplayYMinimum=0.5932  ActiveDisplayYMaximum=0.5951
  Selector : Selector  InputPortWidth=3  IndexOptions=Index vector (dialog)  Indices=[3]  OutputSizes=1
  Selector{1,4,6..7} (4 alike) : Selector  InputPortWidth=3  IndexOptions=Index vector (dialog)  Indices=[2]  OutputSizes=1
  Selector2 : Selector  InputPortWidth=3  IndexOptions=Index vector (dialog)  Indices=[1]  OutputSizes=1
  Selector3 : Selector  InputPortWidth=3  IndexOptions=Index vector (dialog)  Indices=[3]  OutputSizes=1
  Selector5 : Selector  InputPortWidth=3  IndexOptions=Index vector (dialog)  Indices=[1]  OutputSizes=1
  Selector8 : Selector  InputPortWidth=3  IndexOptions=Index vector (dialog)  Indices=[1]  OutputSizes=1
  SinCos : Trigonometry  Operator=sincos
  SinCos1 : Trigonometry  Commented=on  Operator=sincos
  Sqrt : Sqrt
  Square{,1..4} (5 alike) : Math  Operator=square
  Sum{,3..4,6,11..12,17} (7 alike) : Sum
  Sum1 : Sum  Inputs=-+
  Sum{9..10,15,22} (4 alike) : Sum  Inputs=|+-
  Sum{2,7..8,13..14} (5 alike) : Sum  Inputs=+-
  Sum16 : Sum  Commented=on  Inputs=|+-
  Sum18 : Sum  Inputs=|++
  Sum19 : Sum  Inputs=++-
  Sum5 : Sum  Commented=on  Inputs=|+-
  Switch : Switch  Criteria=u2 > Threshold  SaturateOnIntegerOverflow=off  InputSameDT=off
  Switch1 : Switch  Criteria=u2 > Threshold  SaturateOnIntegerOverflow=off  InputSameDT=off
  Tan : Trigonometry  Operator=tan
  Tan1 : Trigonometry
  Tan2 : Trigonometry  Operator=cos
  Tan3 : Trigonometry
  Tan4 : Trigonometry  Operator=cos
  Tan5 : Trigonometry  Operator=tan
  Terminator : Terminator  Commented=on
  Terminator1 : Terminator  Commented=on
  Unit Delay : UnitDelay  Commented=on  SampleTime=-1  HasFrameUpgradeWarning=on
  Roll Cmd : Outport
  Pitch Cmd : Outport  Port=2
  wires:
  Bus Selector1/1 -> Selector4/1, Selector5/1  "<Ve>"
  Lateral velocity/1(el) -> Sum5/2  "vl"
  Cos/1 -> Divide/2
  Divide/1 -> Asin1/1
  From/1 -> Cos/1
  Gain1/1 -> Divide/1
  "Lateral velocity controller "/1 -> Gain1/1
  Selector1/1 -> [Pitch]
  Bus Selector2/1 -> Selector3/1, Selector1/1  "<Euler>"
  Enable/1 -> [Enable]
  Bus Selector3/1 -> Selector6/1, Selector2/1  "<Xe>"
  Yaw Reference/1 -> [yaw_ref], Tan/1
  Tan/1 -> [tan_yaw_ref]
  X Reference/1 -> Sum1/1, Sum/1
  Selector2/1 -> [x_pose]
  [x_pose] -> Sum1/2
  Selector6/1 -> [y_pose]
  [y_pose] -> Sum2/1
  Y Reference/1 -> Sum2/2, Sum3/2
  [tan_yaw_ref] -> Product/1
  Sum2/1 -> Product/2
  Product/1 -> Sum4/2
  Sum1/1 -> Sum4/1
  Sum4/1 -> Divide1/1
  Square/1 -> Sum6/1
  [tan_yaw_ref] -> Square/1
  Sum6/1 -> Divide1/2
  Constant/1 -> Sum6/2
  Product1/1 -> Sum3/1
  [tan_yaw_ref] -> Product1/2
  Divide1/1 -> Sum/2, Product1/1
  [x_pose] -> Sum7/1
  Sum/1 -> Sum7/2
  [yaw_ref] -> Tan1/1
  Sum7/1 -> Product2/1
  Tan1/1 -> Product2/2
  [y_pose] -> Sum8/1
  Sum3/1 -> Sum8/2
  [yaw_ref] -> Tan2/1
  Tan2/1 -> Product3/2
  Sum8/1 -> Product3/1
  Product2/1 -> Sum9/1
  Product3/1 -> Sum9/2
  Constant1/1 -> Sum5/1
  Constant2/1 -> Sum10/1
  Selector5/1 -> [vx]
  Selector4/1 -> [vy]
  Sum9/1 -> [err_track]
  Square1/1 -> Sum11/1
  [tan_yaw_ref] -> Square1/1
  Constant3/1 -> Sum11/2
  Sum11/1 -> Divide2/2
  [vx] -> Sum12/1
  [tan_yaw_ref] -> Product4/2
  Product4/1 -> Sum12/2
  [vy] -> Product4/1
  Sum12/1 -> Divide2/1
  Divide2/1 -> Sum13/2, Product5/1
  [tan_yaw_ref] -> Product5/2
  [vx] -> Sum13/1
  [yaw_ref] -> Tan3/1
  Tan3/1 -> Product6/2
  Sum13/1 -> Product6/1
  Product5/1 -> Sum14/2
  [vy] -> Sum14/1
  [yaw_ref] -> Tan4/1
  Tan4/1 -> Product7/2
  Sum14/1 -> Product7/1
  Product6/1 -> Sum15/1
  Product7/1 -> Sum15/2
  Sum15/1 -> [errdot_track]
  Atan/1 -> Gain6/1
  Unit Delay/1 -> Sum16/2
  Sum16/1 -> Gain/1
  Gain/1 -> Mux/1
  Mux/1 -> Scope/1
  Constant5/1 -> Gain2/1
  Gain2/1 -> Product8/1
  Constant6/1 -> Tan5/1
  Tan5/1 -> Product8/2
  Product8/1 -> Divide3/1
  [vx] -> Square2/1
  Square2/1 -> Sum17/1
  Square3/1 -> Sum17/2
  [vy] -> Square3/1
  Sum17/1 -> Sqrt/1
  Sqrt/1 -> [v_plane]
  [v_plane] -> Max/1
  Max/1 -> Divide3/2
  Constant7/1 -> Max/2
  Divide3/1 -> [wn]
  SinCos1/1 -> Terminator/1
  SinCos1/2 -> Terminator1/1
  [wn] -> Square4/1
  Square4/1 -> Gain3/1
  Gain3/1 -> Product9/1
  Constant8/1 -> Product9/2
  [wn] -> Product11/2
  Gain4/1 -> Product10/1
  Constant9/1 -> Product10/2
  Constant10/1 -> Product11/1
  Product11/1 -> Gain4/1
  Product9/1 -> [Kp]
  Product10/1 -> [Kd]
  Selector3/1 -> [Yaw]  "yaw"
  Bus Selector4/1 -> [Course]  "<course>"
  [err_track] -> Product12/1
  [Kp] -> Product12/2
  [errdot_track] -> Product13/1
  [Kd] -> Product13/2
  Product12/1 -> Sum18/1
  Product13/1 -> Sum18/2
  Sum18/1 -> Divide4/1
  Constant12/1 -> Divide4/2
  Divide4/1 -> Sum19/1
  [yaw_ref] -> Sum19/2
  Switch/1 -> [crs_fdbk]
  [Course] -> Switch/1
  [crs_fdbk] -> Sum19/3
  Compare To Constant/1 -> Switch/2
  [v_plane] -> Compare To Constant/1
  [Yaw] -> Switch/3
  Sum19/1 -> Atan/1
  Gain5/1 -> Display2/1
  Gain6/1 -> Roll Cmd/1
  Mode/1 -> Compare To Constant1/1
  Compare To Constant1/1 -> Switch1/2
  Pitch Reference/1 -> Switch1/3
  Switch1/1 -> Pitch Cmd/1
  SinCos/2 -> Forward velocity/4(cos)
  States/1 -> Bus Selector5/1, Bus Selector6/1, Bus Selector4/1, Bus Selector2/1, Bus Selector1/1, Bus Selector3/1
  Selector/1 -> SinCos/1  "yaw"
  Constant11/1 -> Sum22/1
  Sum22/1 -> Forward velocity controller/1  "e_vx"
  ? -> ?
  Forward velocity controller/1 -> Gain7/1
  Gain7/1 -> Asin/1
  SinCos/1 -> Forward velocity/3(sin)
  Bus Selector6/1 -> Selector/1  "<Euler>"
  Forward velocity/1(ef) -> Sum22/2  "vf"
  Bus Selector5/1 -> Selector7/1, Selector8/1  "<Ve>"
  Selector8/1 -> Forward velocity/2(vx)
  Selector7/1 -> Forward velocity/1(vy)
  Saturation1/1 -> Rate Limiter1/1
  Rate Limiter1/1 -> Gain8/1
  Asin/1 -> Saturation1/1
  Gain8/1 -> Switch1/1

== system VTOLAutopilotController/Low level controller/Multicopter Controller/Horizontal Position Control ==
  note: Forward Motion is controlled using Tilt.
      | Lateral Motion occurs using roll.
  XRef : Inport
  YRef : Inport  Port=2
  States : Inport  Port=3
  Reset : Inport  Port=4
  Enable : EnablePort
  Gain : Gain  Gain=-1
  Rate Limiter : RateLimiter  RisingSlewLimit=controlParams.VTOLmaxRollSlewrate  FallingSlewLimit=controlParams.VTOLminRollSlewrate  SampleTimeMode=inherited
  Rate Limiter1 : RateLimiter  RisingSlewLimit=controlParams.VTOLmaxPitchSlewrate  FallingSlewLimit=controlParams.VTOLminPitchSlewrate  SampleTimeMode=inherited
  Saturation : Saturate  UpperLimit=controlParams.VTOLmaxRoll  LowerLimit=controlParams.VTOLminRoll
  Saturation1 : Saturate  UpperLimit=controlParams.VTOLmaxPitch  LowerLimit=controlParams.VTOLminPitch
  XY Controller : Subsystem
  Roll Cmd : Outport
  Pitch Cmd : Outport  Port=2
  wires:
  XRef/1 -> XY Controller/1(X_ref)
  YRef/1 -> XY Controller/2(Y_ref)
  States/1 -> XY Controller/3(States)
  XY Controller/1(Forward cmd) -> Saturation1/1
  XY Controller/2(Sideward Cmd) -> Saturation/1
  Saturation/1 -> Rate Limiter/1
  Rate Limiter/1 -> Roll Cmd/1
  Saturation1/1 -> Rate Limiter1/1
  Gain/1 -> Pitch Cmd/1
  Rate Limiter1/1 -> Gain/1
  Reset/1 -> XY Controller/4(Reset)

== system VTOLAutopilotController/Low level controller/Multicopter Controller/Organize Inputs ==
  commanded phi torque : Inport
  commanded theta torque : Inport  Port=2
  commanded psi torque : Inport  Port=3
  commanded thrust : Inport  Port=4
  command tilt : Inport  Port=5
  Out Bus Element : Outport  PortName=MixerCommands  Element=w_phi
  Out Bus Element1 : Outport  PortName=MixerCommands  Element=w_theta
  Out Bus Element2 : Outport  PortName=MixerCommands  Element=w_psi
  Out Bus Element3 : Outport  PortName=MixerCommands  Element=w_z
  Out Bus Element4 : Outport  PortName=MixerCommands  Element=w_tilt
  wires:
  commanded theta torque/1 -> Out Bus Element1/1
  commanded thrust/1 -> Out Bus Element3/1
  command tilt/1 -> Out Bus Element4/1
  commanded phi torque/1 -> Out Bus Element/1
  commanded psi torque/1 -> Out Bus Element2/1

== system VTOLAutopilotController/Low level controller/Multicopter Controller/Signal_Fader_OnOff ==
  SW : Inport
  Input_On : Inport  Port=2
  Input_Off : Inport  Port=3
  Fading_Time : Inport  Port=4
  Compare To Constant : simulink/Logic and Bit Operations/Compare To Constant  relop===  const=0  OutDataTypeStr=boolean
  Fader_Off : Subsystem
  Fader_On : Subsystem
  Product : Product
  Product1 : Product
  Sum{,1..3} (4 alike) : Sum  Inputs=+-
  Switch : Switch  Criteria=u2 > Threshold  SaturateOnIntegerOverflow=off  InputSameDT=off
  Switch1 : Switch  Criteria=u2 > Threshold  SaturateOnIntegerOverflow=off  InputSameDT=off
  Switch2 : Switch  Criteria=u2 > Threshold  SaturateOnIntegerOverflow=off  InputSameDT=off
  Unit Delay : UnitDelay  SampleTime=-1  HasFrameUpgradeWarning=on
  Unit Delay1 : UnitDelay  SampleTime=-1  HasFrameUpgradeWarning=on
  Unit Delay2 : UnitDelay  SampleTime=-1  HasFrameUpgradeWarning=on
  Out : Outport
  wires:
  SW/1 -> [Engage]
  Fading_Time/1 -> [Fade_Time]
  [Engage] -> Fader_On/1(SW)
  [Fade_Time] -> Fader_On/2(Fader_Time)
  [Engage] -> Compare To Constant/1
  Compare To Constant/1 -> Fader_Off/1(SW)
  [Fade_Time] -> Fader_Off/2(Fader_Time)
  Input_On/1 -> [On_Input]
  Input_Off/1 -> [Off_Input]
  Unit Delay/1 -> [Out_Capture]
  Switch/1 -> Unit Delay/1, Out/1
  [On_Input] -> Sum/1
  Sum/1 -> Switch/1
  [On_Input] -> Sum1/1
  [Out_Capture] -> Sum1/2
  Sum1/1 -> Switch1/3
  Switch1/1 -> Unit Delay1/1, Product/1
  Unit Delay1/1 -> Switch1/1
  [Engage] -> Switch1/2
  Product/1 -> Sum/2
  Fader_On/1(On) -> Product/2
  [Engage] -> Switch/2
  Sum2/1 -> Switch/3
  Product1/1 -> Sum2/2
  [Off_Input] -> Sum2/1
  [Off_Input] -> Sum3/1
  [Engage] -> Switch2/2
  [Out_Capture] -> Sum3/2
  Sum3/1 -> Switch2/1
  Switch2/1 -> Unit Delay2/1, Product1/2
  Unit Delay2/1 -> Switch2/3
  Fader_Off/1(On) -> Product1/1

== system VTOLAutopilotController/Low level controller/Multicopter Controller/Signal_Fader_OnOff1 ==
  SW : Inport
  Input_On : Inport  Port=2
  Input_Off : Inport  Port=3
  Fading_Time : Inport  Port=4
  Compare To Constant : simulink/Logic and Bit Operations/Compare To Constant  relop===  const=0  OutDataTypeStr=boolean
  Fader_Off : Subsystem
  Fader_On : Subsystem
  Product : Product
  Product1 : Product
  Sum{,1..3} (4 alike) : Sum  Inputs=+-
  Switch : Switch  Criteria=u2 > Threshold  SaturateOnIntegerOverflow=off  InputSameDT=off
  Switch1 : Switch  Criteria=u2 > Threshold  SaturateOnIntegerOverflow=off  InputSameDT=off
  Switch2 : Switch  Criteria=u2 > Threshold  SaturateOnIntegerOverflow=off  InputSameDT=off
  Unit Delay : UnitDelay  SampleTime=-1  HasFrameUpgradeWarning=on
  Unit Delay1 : UnitDelay  SampleTime=-1  HasFrameUpgradeWarning=on
  Unit Delay2 : UnitDelay  SampleTime=-1  HasFrameUpgradeWarning=on
  Out : Outport
  wires:
  SW/1 -> [Engage]
  Fading_Time/1 -> [Fade_Time]
  [Engage] -> Fader_On/1(SW)
  [Fade_Time] -> Fader_On/2(Fader_Time)
  [Engage] -> Compare To Constant/1
  Compare To Constant/1 -> Fader_Off/1(SW)
  [Fade_Time] -> Fader_Off/2(Fader_Time)
  Input_On/1 -> [On_Input]
  Input_Off/1 -> [Off_Input]
  Unit Delay/1 -> [Out_Capture]
  Switch/1 -> Unit Delay/1, Out/1
  [On_Input] -> Sum/1
  Sum/1 -> Switch/1
  [On_Input] -> Sum1/1
  [Out_Capture] -> Sum1/2
  Sum1/1 -> Switch1/3
  Switch1/1 -> Unit Delay1/1, Product/1
  Unit Delay1/1 -> Switch1/1
  [Engage] -> Switch1/2
  Product/1 -> Sum/2
  Fader_On/1(On) -> Product/2
  [Engage] -> Switch/2
  Sum2/1 -> Switch/3
  Product1/1 -> Sum2/2
  [Off_Input] -> Sum2/1
  [Off_Input] -> Sum3/1
  [Engage] -> Switch2/2
  [Out_Capture] -> Sum3/2
  Sum3/1 -> Switch2/1
  Switch2/1 -> Unit Delay2/1, Product1/2
  Unit Delay2/1 -> Switch2/3
  Fader_Off/1(On) -> Product1/1

== system VTOLAutopilotController/Low level controller/Multicopter Controller/Subsystem ==
  inTransition : Inport
  States : Inport  Port=2
  Target : Inport  Port=3
  YawTrack : Inport  Port=4
  Bus Selector : BusSelector  OutputSignals=ypr
  NOT : Logic  Operator=NOT  IconShape=distinctive  AllPortsSameDT=off  OutDataTypeStr=boolean
  Selector : Selector  InputPortWidth=3  IndexOptions=Index vector (dialog)  Indices=[1]  OutputSizes=1
  Switch : Switch  Criteria=u2 > Threshold  SaturateOnIntegerOverflow=off  InputSameDT=off
  Terminator : Terminator
  Triggered Subsystem : Subsystem  TreatAsAtomicUnit=on
  Yaw Reference : Outport
  wires:
  inTransition/1 -> NOT/1, Triggered Subsystem/Trigger
  States/1 -> Bus Selector/1
  Bus Selector/1 -> Selector/1  "<ypr>"
  Selector/1 -> Triggered Subsystem/1(YawHold)
  NOT/1 -> Switch/2
  Switch/1 -> Yaw Reference/1
  Target/1 -> Switch/1
  YawTrack/1 -> Switch/3
  Triggered Subsystem/1(Reference) -> Terminator/1  "Stable"

== system VTOLAutopilotController/Low level controller/Scheduler/FixedWingScheduler ==
  note: C opyright 2024 The MathWorks, Inc.
  note: Fixed Wing Control Mixer
  FlightState : Inport
  FixedWingActuators : Inport  Port=2  OutDataTypeStr=Bus: FixedWingCtrlBus
  TransitionDone : Inport  Port=3
  States : Inport  Port=4
  Bus Selector : BusSelector  OutputSignals=airspeed
  Merge : Merge  Inputs=4
  Switch Case : SwitchCase  CaseConditions={flightState.Hover, flightState.Transition, flightState.FixedWing,flightState.BackTransition}  ShowDefaultCase=off
  Switch Case Action Subsystem : Subsystem  TreatAsAtomicUnit=on
  Switch Case Action Subsystem1 : Subsystem  TreatAsAtomicUnit=on
  Switch Case Action Subsystem2 : Subsystem  TreatAsAtomicUnit=on
  Switch Case Action Subsystem3 : Subsystem  TreatAsAtomicUnit=on
  ActuatorControls : Outport
  wires:
  FlightState/1 -> Switch Case/1
  FixedWingActuators/1 -> Switch Case Action Subsystem3/1(FixedWingActuators), Switch Case Action Subsystem2/1(FixedWingActuators), Switch Case Action Subsystem1/1(FixedWingActuators)
  Switch Case/3 -> Switch Case Action Subsystem2/Action
  Switch Case/2 -> Switch Case Action Subsystem1/Action
  Switch Case Action Subsystem3/1(FixedWingControls) -> Merge/4
  Merge/1 -> ActuatorControls/1
  Switch Case Action Subsystem1/1(FixedWingControls) -> Merge/2
  Switch Case/4 -> Switch Case Action Subsystem3/Action
  Switch Case Action Subsystem/1(FixedWingControls) -> Merge/1
  Switch Case/1 -> Switch Case Action Subsystem/Action
  Switch Case Action Subsystem2/1(FixedWingControls) -> Merge/3
  States/1 -> Bus Selector/1
  Bus Selector/1 -> Switch Case Action Subsystem3/3(airspeed), Switch Case Action Subsystem1/3(airspeed)  "<airspeed>"
  TransitionDone/1 -> Switch Case Action Subsystem3/2(TransitionDone), Switch Case Action Subsystem1/2(TransitionDone)
